simulink model "SIx_pulse_converter"  (R2018b)
settings: Solver=FixedStepAuto  StartTime=0.0  StopTime=1  FixedStep=10e-6  RelTol=1e-3  EnableMultiTasking=on
settings Model: Creator=User  LastModifiedBy=lokes
settings DataIOCC: LimitDataPoints=on  SaveFormat=Array
settings OptimizationCC: LifeSpan=inf
settings DebuggingCC: SolverPrmCheckMsg=warning  SFUnexpectedBacktrackingDiag=warning  SFNoUnconditionalDefaultTransitionDiag=warning  SFExecutionAtInitializationDiag=none
settings HardwareCC: ProdBitPerPointer=32  ProdBitPerSizeT=32  ProdBitPerPtrDiffT=32  ProdLargestAtomicFloat=None  ProdIntDivRoundTo=Undefined  ProdEndianess=Unspecified  ProdWordSize=32  ProdHWDeviceType=32-bit Generic
settings ModelReferenceCC: PropagateSignalLabelsOutOfModel=off
settings SFSimCC: SimUseLocalCustomCode=off
settings RTWCC: RTWUseLocalCustomCode=off
settings CodeAppCC: StateflowObjectComments=on
settings GRTTargetCC: TargetLangStandard=C89/C90 (ANSI)  GeneratePreprocessorConditionals=Disable all
settings ConfigComp: CovMetricSettings=dw  CovHtmlReporting=on  CovSaveCumulativeToWorkspaceVar=on  CovSaveSingleToWorkspaceVar=on  CovExternalEMLEnable=off  CovSFcnEnable=off

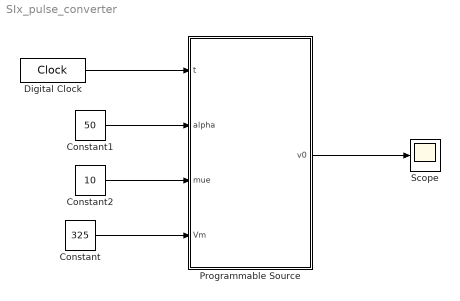
== system SIx_pulse_converter ==
  Constant : Constant  Value=325
  Constant1 : Constant  Value=50
  Constant2 : Constant  Value=10
  Digital Clock : DigitalClock  SampleTime=10e-6
  Programmable Source : MATLAB Function  TreatAsAtomicUnit=on
  Scope : Scope
  wires:
  Digital Clock/1 -> Programmable Source/1(t)
  Constant/1 -> Programmable Source/4(Vm)
  Programmable Source/1(v0) -> Scope/1
  Constant1/1 -> Programmable Source/2(alpha)
  Constant2/1 -> Programmable Source/3(mue)

== matlab function SIx_pulse_converter/Programmable Source ==
  data: t input; v0 output; alpha input; mue input; Vm input
function v0  = fcn(t,alpha,mue,Vm)
%#codegen
% phase angle difference between a and b
f = 50;
w1 = 2*pi*f;  % For variable frequency operation
 w = w1;     % Use it for variable freq operation
%w = 2*pi*50; % For constant frequency operation
%Vm = 325; % Peak of source voltage

alpha = alpha*pi/180;
mue = mue*pi/180;
%
va = Vm*sin(w*t);
vb = Vm*sin((w*t)-(2*pi/3));
vc = Vm*sin((w*t)+(2*pi/3));

vab = va - vb;
vac = va - vc;
vbc = vb - vc;
vba = vb - va;
vca = vc - va;
vcb = vc - vb;

V = [vab, vac, vbc, vba, vca, vcb];

if max(V) == vab         
    if max (vcb, vac) == vcb
        if (alpha+mue) <= pi/6
            if vab <= sqrt(3)*Vm*sin((pi/3)+alpha)
                V0 = vcb;
            elseif  (sqrt(3)*Vm*sin((pi/3)+alpha) < vab) &&  (vab <= sqrt(3)*Vm*sin((pi/3)+alpha+mue))   
                V0 = -3*vb/2;
            else
                V0 = vab;
            end
        else
            if alpha <= pi/6
                if vab <= sqrt(3)*Vm*sin((pi/3)+alpha)
                    V0 = vcb;
                else    
                    V0 = -3*vb/2;
                end
            else
                V0 = vcb;
            end
        end
    else
        if (alpha+mue) <= pi/6
            V0 = vab;
        else
            if alpha <= pi/6
                if vab >= sqrt(3)*Vm*sin((pi/3)+alpha+mue)
                    V0 = -3*vb/2;
                else
                    V0 = vab;
                end
            else
                if vab >= sqrt(3)*Vm*sin((pi/3)+alpha)
                    V0 = vcb;
                elseif  (sqrt(3)*Vm*sin((pi/3)+alpha) > vab) &&  (vab >= sqrt(3)*Vm*sin((pi/3)+alpha+mue))   
                    V0 = -3*vb/2;
                else
                    V0 = vab;
                end
            end
        end
    end

    
    
    
elseif max(V) == vac
    if max (vab, vbc) == vab
        if (alpha+mue) <= pi/6
            if vac <= sqrt(3)*Vm*sin((pi/3)+alpha) 
                V0 = vab;
            elseif (sqrt(3)*Vm*sin((pi/3)+alpha) < vac) && (vac <= sqrt(3)*Vm*sin((pi/3)+alpha+mue))
                V0 = 3*va/2;
            else
                V0 = vac;
            end
        else
            if alpha <= pi/6
                if vac <= sqrt(3)*Vm*sin((pi/3)+alpha)
                    V0 = vab;
                else    
                    V0 = 3*va/2;
                end
            else
                V0 = vab;
            end
        end
    else
        if (alpha+mue) <= pi/6
            V0 = vac;
        else
            if alpha <= pi/6
                if vac >= sqrt(3)*Vm*sin((pi/3)+alpha+mue)
                    V0 = 3*va/2;
                else
                    V0 = vac;
                end
            else
                if vac >= sqrt(3)*Vm*sin((pi/3)+alpha)
                    V0 = vab;
                elseif  (sqrt(3)*Vm*sin((pi/3)+alpha) > vac) &&  (vac >= sqrt(3)*Vm*sin((pi/3)+alpha+mue))   
                    V0 = 3*va/2;
                else
                    V0 = vac;
                end
            end
        end
    end
 
    
    
    
    
elseif max(V) == vbc
    if max (vac, vba) == vac
        if (alpha+mue) <= pi/6
            if vbc <= sqrt(3)*Vm*sin((pi/3)+alpha) 
                V0 = vac;
            elseif (sqrt(3)*Vm*sin((pi/3)+alpha) < vbc) && (vbc <= sqrt(3)*Vm*sin((pi/3)+alpha+mue))
                V0 = -3*vc/2;
            else
                V0 = vbc;
            end
        else
            if alpha <= pi/6
                if vbc <= sqrt(3)*Vm*sin((pi/3)+alpha)
                    V0 = vac;
                else    
                    V0 = -3*vc/2;
                end
            else
                V0 = vac;
            end
        end
            
    else
        if (alpha+mue) <= pi/6
            V0 = vbc;
        else
            if alpha <= pi/6
                if vbc >= sqrt(3)*Vm*sin((pi/3)+alpha+mue)
                    V0 = -3*vc/2;
                else
                    V0 = vbc;
                end
            else
                if vbc >= sqrt(3)*Vm*sin((pi/3)+alpha)
                    V0 = vac;
                elseif  (sqrt(3)*Vm*sin((pi/3)+alpha) > vbc) &&  (vbc >= sqrt(3)*Vm*sin((pi/3)+alpha+mue))   
                    V0 = -3*vc/2;
                else
                    V0 = vbc;
                end
            end
        end
    end

    
  
    
 
        
elseif max(V) == vba
    if max (vbc, vca) == vbc
        if (alpha+mue) <= pi/6
            if vba <= sqrt(3)*Vm*sin((pi/3)+alpha) 
                V0 = vbc;
            elseif (sqrt(3)*Vm*sin((pi/3)+alpha) < vba) && (vba <= sqrt(3)*Vm*sin((pi/3)+alpha+mue))
                V0 = 3*vb/2;
            else
                V0 = vba;
            end
        else
            if alpha <= pi/6
                if vba <= sqrt(3)*Vm*sin((pi/3)+alpha)
                    V0 = vbc;
                else    
                    V0 = 3*vb/2;
                end
            else
                V0 = vbc;
            end
        end
    else
        if (alpha+mue) <= pi/6
            V0 = vba;
         else
            if alpha <= pi/6
                if vba >= sqrt(3)*Vm*sin((pi/3)+alpha+mue)
                    V0 = 3*vb/2;
                else
                    V0 = vba;
                end
            else
                if vba >= sqrt(3)*Vm*sin((pi/3)+alpha)
                    V0 = vbc;
                elseif  (sqrt(3)*Vm*sin((pi/3)+alpha) > vba) &&  (vba >= sqrt(3)*Vm*sin((pi/3)+alpha+mue))   
                    V0 = 3*vb/2;
                else
                    V0 = vba;
                end
            end
        end   
    end 
        
 
    
    
elseif max(V) == vca
    if max (vba, vcb) == vba
        if (alpha+mue) <= pi/6
            if vca <= sqrt(3)*Vm*sin((pi/3)+alpha) 
                V0 = vba;
            elseif (sqrt(3)*Vm*sin((pi/3)+alpha) < vca) && (vca <= sqrt(3)*Vm*sin((pi/3)+alpha+mue))
                V0 = -3*va/2;
            else
                V0 = vca;
            end
        else
            if alpha <= pi/6
                if vca <= sqrt(3)*Vm*sin((pi/3)+alpha)
                    V0 = vba;
                else    
                    V0 = -3*va/2;
                end
            else
                V0 = vba;
            end
        end
        
    else
        if (alpha+mue) <= pi/6
            V0 = vca;
        else
            if alpha <= pi/6
                if vca >= sqrt(3)*Vm*sin((pi/3)+alpha+mue)
                    V0 = -3*va/2;
                else
                    V0 = vca;
                end
            else
                if vca >= sqrt(3)*Vm*sin((pi/3)+alpha)
                    V0 = vba;
                elseif  (sqrt(3)*Vm*sin((pi/3)+alpha) > vca) &&  (vca >= sqrt(3)*Vm*sin((pi/3)+alpha+mue))   
                    V0 = -3*va/2;
                else
                    V0 = vca;
                end
            end
        end
    end 
    
    
    
    
    
elseif max(V) == vcb
    if max (vca, vab) == vca
        if (alpha+mue) <= pi/6
            if vcb <= sqrt(3)*Vm*sin((pi/3)+alpha) 
                V0 = vca;
            elseif (sqrt(3)*Vm*sin((pi/3)+alpha) < vcb) && (vcb <= sqrt(3)*Vm*sin((pi/3)+alpha+mue))
                V0 = 3*vc/2;
            else
                V0 = vcb;
            end
        else
            if alpha <= pi/6
                if vcb <= sqrt(3)*Vm*sin((pi/3)+alpha)
                    V0 = vca;
                else    
                    V0 = 3*vc/2;
                end
            else
                V0 = vca;
            end
        end
    else
        if (alpha+mue) <= pi/6
            V0 = vcb;
        else
            if alpha <= pi/6
                if vcb >= sqrt(3)*Vm*sin((pi/3)+alpha+mue)
                    V0 = 3*vc/2;
                else
                    V0 = vcb;
                end
            else
                if vcb >= sqrt(3)*Vm*sin((pi/3)+alpha)
                    V0 = vca;
                elseif  (sqrt(3)*Vm*sin((pi/3)+alpha) > vcb) &&  (vcb >= sqrt(3)*Vm*sin((pi/3)+alpha+mue))   
                    V0 = 3*vc/2;
                else
                    V0 = vcb;
                end
            end
        end
    end 
    
    
    
else
    V0 = va;
    
end
%}

v0 = V0;
